simulink model "poco_ref_al_r307"  (Simulink 6.2)
settings: Solver=ode45  StartTime=0.0  StopTime=100000  RelTol=1e-3
libraries: xbsIndex_r3 x1012, xps_library x42, ddc_library x4, adcscope_lib x2, fft_library x2, pfb_library x2, delay_lib x1
(part 6 of 9)

== system poco_ref_al_r307/dir_x/bb ==
  a+bi : Inport  Port=1  LatchInput=off
  c+di : Inport  Port=2  LatchInput=off
  new_acc : Inport  Port=3  LatchInput=off
  Counter : xbsIndex_r3/Counter  cnt_type=Free Running  n_bits=11  bin_pt=0  arith_type=Unsigned  start_count=0  cnt_to=Inf  cnt_by_val=1  operation=Up  explicit_period=off  period=1  load_pin=off  rst=on  en=on  dbl_ovrd=off  show_param=off  use_rpm=on  gen_core=off
      settings: xl_area=[0, 0, 0, 0, 0, 0, 0]
  Delay3 : xbsIndex_r3/Delay  latency=5  reg_retiming=off  explicit_period=off  period=1  en=off  accept_only_valid=off  init_zero=on  dbl_ovrd=off  show_param=off
      settings: xl_area=[0, 0, 0, 0, 0, 0, 0]
  Reinterpret : xbsIndex_r3/Reinterpret  force_arith_type=on  arith_type=Unsigned  force_bin_pt=on  bin_pt=0  force_valid=on
  c_to_ri : Subsystem  mask(Complex to Real-Imag){n_bits=4, bin_pt=3}
      mask prompts: n_bits "Bit Width"; bin_pt "Binary Point"
      mask help: Outputs real and imaginary components of a complex input.
      mask init:
      | annotation=sprintf('%d_%d r/i',n_bits,bin_pt);
      | set_param(gcb,'AttributesFormatString',annotation);
      settings: AttributesFormatString=4_3 r/i
      mask Help:
      | <pre>
      | Description::
      | 
      | Outputs real and imaginary components of a complex input.
      | Useful for simplifying interconnects.
      | See also: Real-Imag to Complex (ri_to_c)
      | 
      | Mask Parameters::
      | 
      | Bit Width (n_bits): Specifies the width of the real/imaginary components.
      | Assumed equal for both components.
      | 
      | Binary Point (bin_pt): Specifies the binary point location in the real/imaginary components.
      | Assumed equal for both components.
      | </pre>
  c_to_ri1 : Subsystem  mask(Complex to Real-Imag){n_bits=4, bin_pt=3}
      mask prompts: n_bits "Bit Width"; bin_pt "Binary Point"
      mask help: Outputs real and imaginary components of a complex input.
      mask init:
      | annotation=sprintf('%d_%d r/i',n_bits,bin_pt);
      | set_param(gcb,'AttributesFormatString',annotation);
      settings: AttributesFormatString=4_3 r/i
      mask Help:
      | <pre>
      | Description::
      | 
      | Outputs real and imaginary components of a complex input.
      | Useful for simplifying interconnects.
      | See also: Real-Imag to Complex (ri_to_c)
      | 
      | Mask Parameters::
      | 
      | Bit Width (n_bits): Specifies the width of the real/imaginary components.
      | Assumed equal for both components.
      | 
      | Binary Point (bin_pt): Specifies the binary point location in the real/imaginary components.
      | Assumed equal for both components.
      | </pre>
  cmult_4bit_br* : Subsystem  mask(cmult_4bit_br*){mult_latency=3, add_latency=2}
      mask prompts: mult_latency "Mult Latency"; add_latency "Add Latency"
      mask help: Perform a conjugating complex multiplication (a+bi)(c-di)=(ac+bd)+(bc-ad)i. Implements the logic in Block RAM.
      mask Help: eval('xlWeb([getenv(''MLIB_ROOT''), ''\doc\html\sp_cmult_4bit_br_\sp_cmult_4bit_br_.html''])')
  real : xps_library/Shared BRAM  Tag=xps:bram  arith_type=Unsigned  addr_width=chan_bits+1  data_width=32  data_bin_pt=0  init_vals=0  sample_rate=1
  vacc_32bit : Subsystem  mask{n_chans=n_chans}
      mask prompts: n_chans "Number of channels"
      mask init:
      | chan_bits=ceil(log2(n_chans));
  wires:
  cmult_4bit_br*/1(real) -> vacc_32bit/1(din)
  new_acc/1 -> Delay3/1
  vacc_32bit/1(dout) -> Reinterpret/1
  c_to_ri/1(re) -> cmult_4bit_br*/1(a)
  c_to_ri/2(im) -> cmult_4bit_br*/2(b)
  c_to_ri1/1(re) -> cmult_4bit_br*/3(c)
  c_to_ri1/2(im) -> cmult_4bit_br*/4(d)
  a+bi/1 -> c_to_ri/1(c)
  c+di/1 -> c_to_ri1/1(c)
  Delay3/1 -> Counter/1, vacc_32bit/2(new_acc)
  vacc_32bit/2(valid) -> real/3, Counter/2
  Counter/1 -> real/1
  Reinterpret/1 -> real/2

== system poco_ref_al_r307/dir_x/bc ==
  a+bi : Inport  Port=1  LatchInput=off
  c+di : Inport  Port=2  LatchInput=off
  new_acc : Inport  Port=3  LatchInput=off
  Counter : xbsIndex_r3/Counter  cnt_type=Free Running  n_bits=11  bin_pt=0  arith_type=Unsigned  start_count=0  cnt_to=Inf  cnt_by_val=1  operation=Up  explicit_period=off  period=1  load_pin=off  rst=on  en=on  dbl_ovrd=off  show_param=off  use_rpm=on  gen_core=off
      settings: xl_area=[0, 0, 0, 0, 0, 0, 0]
  Delay3 : xbsIndex_r3/Delay  latency=5  reg_retiming=off  explicit_period=off  period=1  en=off  accept_only_valid=off  init_zero=on  dbl_ovrd=off  show_param=off
      settings: xl_area=[0, 0, 0, 0, 0, 0, 0]
  Reinterpret : xbsIndex_r3/Reinterpret  force_arith_type=on  arith_type=Unsigned  force_bin_pt=on  bin_pt=0  force_valid=on
  Reinterpret1 : xbsIndex_r3/Reinterpret  force_arith_type=on  arith_type=Unsigned  force_bin_pt=on  bin_pt=0  force_valid=on
  c_to_ri : Subsystem  mask(Complex to Real-Imag){n_bits=4, bin_pt=3}
      mask prompts: n_bits "Bit Width"; bin_pt "Binary Point"
      mask help: Outputs real and imaginary components of a complex input.
      mask init:
      | annotation=sprintf('%d_%d r/i',n_bits,bin_pt);
      | set_param(gcb,'AttributesFormatString',annotation);
      settings: AttributesFormatString=4_3 r/i
      mask Help:
      | <pre>
      | Description::
      | 
      | Outputs real and imaginary components of a complex input.
      | Useful for simplifying interconnects.
      | See also: Real-Imag to Complex (ri_to_c)
      | 
      | Mask Parameters::
      | 
      | Bit Width (n_bits): Specifies the width of the real/imaginary components.
      | Assumed equal for both components.
      | 
      | Binary Point (bin_pt): Specifies the binary point location in the real/imaginary components.
      | Assumed equal for both components.
      | </pre>
  c_to_ri1 : Subsystem  mask(Complex to Real-Imag){n_bits=4, bin_pt=3}
      mask prompts: n_bits "Bit Width"; bin_pt "Binary Point"
      mask help: Outputs real and imaginary components of a complex input.
      mask init:
      | annotation=sprintf('%d_%d r/i',n_bits,bin_pt);
      | set_param(gcb,'AttributesFormatString',annotation);
      settings: AttributesFormatString=4_3 r/i
      mask Help:
      | <pre>
      | Description::
      | 
      | Outputs real and imaginary components of a complex input.
      | Useful for simplifying interconnects.
      | See also: Real-Imag to Complex (ri_to_c)
      | 
      | Mask Parameters::
      | 
      | Bit Width (n_bits): Specifies the width of the real/imaginary components.
      | Assumed equal for both components.
      | 
      | Binary Point (bin_pt): Specifies the binary point location in the real/imaginary components.
      | Assumed equal for both components.
      | </pre>
  cmult_4bit_sl* : Subsystem  mask(cmult_4bit_sl*){mult_latency=3, add_latency=2}
      mask prompts: mult_latency "Mult Latency"; add_latency "Add Latency"
      mask help: Perform a conjugating complex multiplication (a+bi)(c-di)=(ac+bd)+(bc-ad)i. Implements the logic in Slices.
      mask Help: eval('xlWeb([getenv(''MLIB_ROOT''), ''\doc\html\sp_cmult_4bit_sl_\sp_cmult_4bit_sl_.html''])')
  imag : xps_library/Shared BRAM  Tag=xps:bram  arith_type=Unsigned  addr_width=chan_bits+1  data_width=32  data_bin_pt=0  init_vals=0  sample_rate=1
  real : xps_library/Shared BRAM  Tag=xps:bram  arith_type=Unsigned  addr_width=chan_bits+1  data_width=32  data_bin_pt=0  init_vals=0  sample_rate=1
  vacc_0 : Subsystem  mask{n_chans=n_chans}
      mask prompts: n_chans "Number of channels"
      mask init:
      | chan_bits=ceil(log2(n_chans));
  vacc_1 : Subsystem  mask{n_chans=n_chans}
      mask prompts: n_chans "Number of channels"
      mask init:
      | chan_bits=ceil(log2(n_chans));
  wires:
  Counter/1 -> real/1, imag/1
  vacc_1/1(dout) -> Reinterpret1/1
  Reinterpret1/1 -> imag/2
  vacc_1/2(valid) -> imag/3
  Reinterpret/1 -> real/2
  vacc_0/2(valid) -> real/3, Counter/2
  vacc_0/1(dout) -> Reinterpret/1
  new_acc/1 -> Delay3/1
  Delay3/1 -> Counter/1, vacc_0/2(new_acc), vacc_1/2(new_acc)
  c+di/1 -> c_to_ri1/1(c)
  a+bi/1 -> c_to_ri/1(c)
  c_to_ri1/2(im) -> cmult_4bit_sl*/4(d)
  c_to_ri1/1(re) -> cmult_4bit_sl*/3(c)
  c_to_ri/2(im) -> cmult_4bit_sl*/2(b)
  c_to_ri/1(re) -> cmult_4bit_sl*/1(a)
  cmult_4bit_sl*/2(imag) -> vacc_1/1(din)
  cmult_4bit_sl*/1(real) -> vacc_0/1(din)

== system poco_ref_al_r307/dir_x/bd ==
  a+bi : Inport  Port=1  LatchInput=off
  c+di : Inport  Port=2  LatchInput=off
  new_acc : Inport  Port=3  LatchInput=off
  Counter : xbsIndex_r3/Counter  cnt_type=Free Running  n_bits=11  bin_pt=0  arith_type=Unsigned  start_count=0  cnt_to=Inf  cnt_by_val=1  operation=Up  explicit_period=off  period=1  load_pin=off  rst=on  en=on  dbl_ovrd=off  show_param=off  use_rpm=on  gen_core=off
      settings: xl_area=[0, 0, 0, 0, 0, 0, 0]
  Delay3 : xbsIndex_r3/Delay  latency=5  reg_retiming=off  explicit_period=off  period=1  en=off  accept_only_valid=off  init_zero=on  dbl_ovrd=off  show_param=off
      settings: xl_area=[0, 0, 0, 0, 0, 0, 0]
  Reinterpret : xbsIndex_r3/Reinterpret  force_arith_type=on  arith_type=Unsigned  force_bin_pt=on  bin_pt=0  force_valid=on
  Reinterpret1 : xbsIndex_r3/Reinterpret  force_arith_type=on  arith_type=Unsigned  force_bin_pt=on  bin_pt=0  force_valid=on
  c_to_ri : Subsystem  mask(Complex to Real-Imag){n_bits=4, bin_pt=3}
      mask prompts: n_bits "Bit Width"; bin_pt "Binary Point"
      mask help: Outputs real and imaginary components of a complex input.
      mask init:
      | annotation=sprintf('%d_%d r/i',n_bits,bin_pt);
      | set_param(gcb,'AttributesFormatString',annotation);
      settings: AttributesFormatString=4_3 r/i
      mask Help:
      | <pre>
      | Description::
      | 
      | Outputs real and imaginary components of a complex input.
      | Useful for simplifying interconnects.
      | See also: Real-Imag to Complex (ri_to_c)
      | 
      | Mask Parameters::
      | 
      | Bit Width (n_bits): Specifies the width of the real/imaginary components.
      | Assumed equal for both components.
      | 
      | Binary Point (bin_pt): Specifies the binary point location in the real/imaginary components.
      | Assumed equal for both components.
      | </pre>
  c_to_ri1 : Subsystem  mask(Complex to Real-Imag){n_bits=4, bin_pt=3}
      mask prompts: n_bits "Bit Width"; bin_pt "Binary Point"
      mask help: Outputs real and imaginary components of a complex input.
      mask init:
      | annotation=sprintf('%d_%d r/i',n_bits,bin_pt);
      | set_param(gcb,'AttributesFormatString',annotation);
      settings: AttributesFormatString=4_3 r/i
      mask Help:
      | <pre>
      | Description::
      | 
      | Outputs real and imaginary components of a complex input.
      | Useful for simplifying interconnects.
      | See also: Real-Imag to Complex (ri_to_c)
      | 
      | Mask Parameters::
      | 
      | Bit Width (n_bits): Specifies the width of the real/imaginary components.
      | Assumed equal for both components.
      | 
      | Binary Point (bin_pt): Specifies the binary point location in the real/imaginary components.
      | Assumed equal for both components.
      | </pre>
  cmult_4bit_sl* : Subsystem  mask(cmult_4bit_sl*){mult_latency=3, add_latency=2}
      mask prompts: mult_latency "Mult Latency"; add_latency "Add Latency"
      mask help: Perform a conjugating complex multiplication (a+bi)(c-di)=(ac+bd)+(bc-ad)i. Implements the logic in Slices.
      mask Help: eval('xlWeb([getenv(''MLIB_ROOT''), ''\doc\html\sp_cmult_4bit_sl_\sp_cmult_4bit_sl_.html''])')
  imag : xps_library/Shared BRAM  Tag=xps:bram  arith_type=Unsigned  addr_width=chan_bits+1  data_width=32  data_bin_pt=0  init_vals=0  sample_rate=1
  real : xps_library/Shared BRAM  Tag=xps:bram  arith_type=Unsigned  addr_width=chan_bits+1  data_width=32  data_bin_pt=0  init_vals=0  sample_rate=1
  vacc_0 : Subsystem  mask{n_chans=n_chans}
      mask prompts: n_chans "Number of channels"
      mask init:
      | chan_bits=ceil(log2(n_chans));
  vacc_1 : Subsystem  mask{n_chans=n_chans}
      mask prompts: n_chans "Number of channels"
      mask init:
      | chan_bits=ceil(log2(n_chans));
  wires:
  cmult_4bit_sl*/1(real) -> vacc_0/1(din)
  cmult_4bit_sl*/2(imag) -> vacc_1/1(din)
  c_to_ri/1(re) -> cmult_4bit_sl*/1(a)
  c_to_ri/2(im) -> cmult_4bit_sl*/2(b)
  c_to_ri1/1(re) -> cmult_4bit_sl*/3(c)
  c_to_ri1/2(im) -> cmult_4bit_sl*/4(d)
  a+bi/1 -> c_to_ri/1(c)
  c+di/1 -> c_to_ri1/1(c)
  Delay3/1 -> Counter/1, vacc_0/2(new_acc), vacc_1/2(new_acc)
  new_acc/1 -> Delay3/1
  vacc_0/1(dout) -> Reinterpret/1
  vacc_0/2(valid) -> Counter/2, real/3
  Reinterpret/1 -> real/2
  vacc_1/2(valid) -> imag/3
  Reinterpret1/1 -> imag/2
  vacc_1/1(dout) -> Reinterpret1/1
  Counter/1 -> imag/1, real/1

== system poco_ref_al_r307/dir_x/cc ==
  a+bi : Inport  Port=1  LatchInput=off
  c+di : Inport  Port=2  LatchInput=off
  new_acc : Inport  Port=3  LatchInput=off
  Counter : xbsIndex_r3/Counter  cnt_type=Free Running  n_bits=11  bin_pt=0  arith_type=Unsigned  start_count=0  cnt_to=Inf  cnt_by_val=1  operation=Up  explicit_period=off  period=1  load_pin=off  rst=on  en=on  dbl_ovrd=off  show_param=off  use_rpm=on  gen_core=off
      settings: xl_area=[0, 0, 0, 0, 0, 0, 0]
  Delay3 : xbsIndex_r3/Delay  latency=5  reg_retiming=off  explicit_period=off  period=1  en=off  accept_only_valid=off  init_zero=on  dbl_ovrd=off  show_param=off
      settings: xl_area=[0, 0, 0, 0, 0, 0, 0]
  Reinterpret : xbsIndex_r3/Reinterpret  force_arith_type=on  arith_type=Unsigned  force_bin_pt=on  bin_pt=0  force_valid=on
  c_to_ri : Subsystem  mask(Complex to Real-Imag){n_bits=4, bin_pt=3}
      mask prompts: n_bits "Bit Width"; bin_pt "Binary Point"
      mask help: Outputs real and imaginary components of a complex input.
      mask init:
      | annotation=sprintf('%d_%d r/i',n_bits,bin_pt);
      | set_param(gcb,'AttributesFormatString',annotation);
      settings: AttributesFormatString=4_3 r/i
      mask Help:
      | <pre>
      | Description::
      | 
      | Outputs real and imaginary components of a complex input.
      | Useful for simplifying interconnects.
      | See also: Real-Imag to Complex (ri_to_c)
      | 
      | Mask Parameters::
      | 
      | Bit Width (n_bits): Specifies the width of the real/imaginary components.
      | Assumed equal for both components.
      | 
      | Binary Point (bin_pt): Specifies the binary point location in the real/imaginary components.
      | Assumed equal for both components.
      | </pre>
  c_to_ri1 : Subsystem  mask(Complex to Real-Imag){n_bits=4, bin_pt=3}
      mask prompts: n_bits "Bit Width"; bin_pt "Binary Point"
      mask help: Outputs real and imaginary components of a complex input.
      mask init:
      | annotation=sprintf('%d_%d r/i',n_bits,bin_pt);
      | set_param(gcb,'AttributesFormatString',annotation);
      settings: AttributesFormatString=4_3 r/i
      mask Help:
      | <pre>
      | Description::
      | 
      | Outputs real and imaginary components of a complex input.
      | Useful for simplifying interconnects.
      | See also: Real-Imag to Complex (ri_to_c)
      | 
      | Mask Parameters::
      | 
      | Bit Width (n_bits): Specifies the width of the real/imaginary components.
      | Assumed equal for both components.
      | 
      | Binary Point (bin_pt): Specifies the binary point location in the real/imaginary components.
      | Assumed equal for both components.
      | </pre>
  cmult_4bit_br* : Subsystem  mask(cmult_4bit_br*){mult_latency=3, add_latency=2}
      mask prompts: mult_latency "Mult Latency"; add_latency "Add Latency"
      mask help: Perform a conjugating complex multiplication (a+bi)(c-di)=(ac+bd)+(bc-ad)i. Implements the logic in Block RAM.
      mask Help: eval('xlWeb([getenv(''MLIB_ROOT''), ''\doc\html\sp_cmult_4bit_br_\sp_cmult_4bit_br_.html''])')
  real : xps_library/Shared BRAM  Tag=xps:bram  arith_type=Unsigned  addr_width=chan_bits+1  data_width=32  data_bin_pt=0  init_vals=0  sample_rate=1
  vacc_32bit : Subsystem  mask{n_chans=n_chans}
      mask prompts: n_chans "Number of channels"
      mask init:
      | chan_bits=ceil(log2(n_chans));
  wires:
  Reinterpret/1 -> real/2
  Counter/1 -> real/1
  vacc_32bit/2(valid) -> Counter/2, real/3
  Delay3/1 -> Counter/1, vacc_32bit/2(new_acc)
  c+di/1 -> c_to_ri1/1(c)
  a+bi/1 -> c_to_ri/1(c)
  c_to_ri1/2(im) -> cmult_4bit_br*/4(d)
  c_to_ri1/1(re) -> cmult_4bit_br*/3(c)
  c_to_ri/2(im) -> cmult_4bit_br*/2(b)
  c_to_ri/1(re) -> cmult_4bit_br*/1(a)
  vacc_32bit/1(dout) -> Reinterpret/1
  new_acc/1 -> Delay3/1
  cmult_4bit_br*/1(real) -> vacc_32bit/1(din)

== system poco_ref_al_r307/dir_x/cd ==
  a+bi : Inport  Port=1  LatchInput=off
  c+di : Inport  Port=2  LatchInput=off
  new_acc : Inport  Port=3  LatchInput=off
  Counter : xbsIndex_r3/Counter  cnt_type=Free Running  n_bits=11  bin_pt=0  arith_type=Unsigned  start_count=0  cnt_to=Inf  cnt_by_val=1  operation=Up  explicit_period=off  period=1  load_pin=off  rst=on  en=on  dbl_ovrd=off  show_param=off  use_rpm=on  gen_core=off
      settings: xl_area=[0, 0, 0, 0, 0, 0, 0]
  Delay3 : xbsIndex_r3/Delay  latency=5  reg_retiming=off  explicit_period=off  period=1  en=off  accept_only_valid=off  init_zero=on  dbl_ovrd=off  show_param=off
      settings: xl_area=[0, 0, 0, 0, 0, 0, 0]
  Reinterpret : xbsIndex_r3/Reinterpret  force_arith_type=on  arith_type=Unsigned  force_bin_pt=on  bin_pt=0  force_valid=on
  Reinterpret1 : xbsIndex_r3/Reinterpret  force_arith_type=on  arith_type=Unsigned  force_bin_pt=on  bin_pt=0  force_valid=on
  c_to_ri : Subsystem  mask(Complex to Real-Imag){n_bits=4, bin_pt=3}
      mask prompts: n_bits "Bit Width"; bin_pt "Binary Point"
      mask help: Outputs real and imaginary components of a complex input.
      mask init:
      | annotation=sprintf('%d_%d r/i',n_bits,bin_pt);
      | set_param(gcb,'AttributesFormatString',annotation);
      settings: AttributesFormatString=4_3 r/i
      mask Help:
      | <pre>
      | Description::
      | 
      | Outputs real and imaginary components of a complex input.
      | Useful for simplifying interconnects.
      | See also: Real-Imag to Complex (ri_to_c)
      | 
      | Mask Parameters::
      | 
      | Bit Width (n_bits): Specifies the width of the real/imaginary components.
      | Assumed equal for both components.
      | 
      | Binary Point (bin_pt): Specifies the binary point location in the real/imaginary components.
      | Assumed equal for both components.
      | </pre>
  c_to_ri1 : Subsystem  mask(Complex to Real-Imag){n_bits=4, bin_pt=3}
      mask prompts: n_bits "Bit Width"; bin_pt "Binary Point"
      mask help: Outputs real and imaginary components of a complex input.
      mask init:
      | annotation=sprintf('%d_%d r/i',n_bits,bin_pt);
      | set_param(gcb,'AttributesFormatString',annotation);
      settings: AttributesFormatString=4_3 r/i
      mask Help:
      | <pre>
      | Description::
      | 
      | Outputs real and imaginary components of a complex input.
      | Useful for simplifying interconnects.
      | See also: Real-Imag to Complex (ri_to_c)
      | 
      | Mask Parameters::
      | 
      | Bit Width (n_bits): Specifies the width of the real/imaginary components.
      | Assumed equal for both components.
      | 
      | Binary Point (bin_pt): Specifies the binary point location in the real/imaginary components.
      | Assumed equal for both components.
      | </pre>
  cmult_4bit_sl* : Subsystem  mask(cmult_4bit_sl*){mult_latency=3, add_latency=2}
      mask prompts: mult_latency "Mult Latency"; add_latency "Add Latency"
      mask help: Perform a conjugating complex multiplication (a+bi)(c-di)=(ac+bd)+(bc-ad)i. Implements the logic in Slices.
      mask Help: eval('xlWeb([getenv(''MLIB_ROOT''), ''\doc\html\sp_cmult_4bit_sl_\sp_cmult_4bit_sl_.html''])')
  imag : xps_library/Shared BRAM  Tag=xps:bram  arith_type=Unsigned  addr_width=chan_bits+1  data_width=32  data_bin_pt=0  init_vals=0  sample_rate=1
  real : xps_library/Shared BRAM  Tag=xps:bram  arith_type=Unsigned  addr_width=chan_bits+1  data_width=32  data_bin_pt=0  init_vals=0  sample_rate=1
  vacc_0 : Subsystem  mask{n_chans=n_chans}
      mask prompts: n_chans "Number of channels"
      mask init:
      | chan_bits=ceil(log2(n_chans));
  vacc_1 : Subsystem  mask{n_chans=n_chans}
      mask prompts: n_chans "Number of channels"
      mask init:
      | chan_bits=ceil(log2(n_chans));
  wires:
  Counter/1 -> real/1, imag/1
  vacc_1/1(dout) -> Reinterpret1/1
  Reinterpret1/1 -> imag/2
  vacc_1/2(valid) -> imag/3
  Reinterpret/1 -> real/2
  vacc_0/2(valid) -> real/3, Counter/2
  vacc_0/1(dout) -> Reinterpret/1
  new_acc/1 -> Delay3/1
  Delay3/1 -> Counter/1, vacc_0/2(new_acc), vacc_1/2(new_acc)
  c+di/1 -> c_to_ri1/1(c)
  a+bi/1 -> c_to_ri/1(c)
  c_to_ri1/2(im) -> cmult_4bit_sl*/4(d)
  c_to_ri1/1(re) -> cmult_4bit_sl*/3(c)
  c_to_ri/2(im) -> cmult_4bit_sl*/2(b)
  c_to_ri/1(re) -> cmult_4bit_sl*/1(a)
  cmult_4bit_sl*/2(imag) -> vacc_1/1(din)
  cmult_4bit_sl*/1(real) -> vacc_0/1(din)

== system poco_ref_al_r307/dir_x/dd ==
  a+bi : Inport  Port=1  LatchInput=off
  c+di : Inport  Port=2  LatchInput=off
  new_acc : Inport  Port=3  LatchInput=off
  Counter : xbsIndex_r3/Counter  cnt_type=Free Running  n_bits=11  bin_pt=0  arith_type=Unsigned  start_count=0  cnt_to=Inf  cnt_by_val=1  operation=Up  explicit_period=off  period=1  load_pin=off  rst=on  en=on  dbl_ovrd=off  show_param=off  use_rpm=on  gen_core=off
      settings: xl_area=[0, 0, 0, 0, 0, 0, 0]
  Delay3 : xbsIndex_r3/Delay  latency=5  reg_retiming=off  explicit_period=off  period=1  en=off  accept_only_valid=off  init_zero=on  dbl_ovrd=off  show_param=off
      settings: xl_area=[0, 0, 0, 0, 0, 0, 0]
  Reinterpret : xbsIndex_r3/Reinterpret  force_arith_type=on  arith_type=Unsigned  force_bin_pt=on  bin_pt=0  force_valid=on
  c_to_ri : Subsystem  mask(Complex to Real-Imag){n_bits=4, bin_pt=3}
      mask prompts: n_bits "Bit Width"; bin_pt "Binary Point"
      mask help: Outputs real and imaginary components of a complex input.
      mask init:
      | annotation=sprintf('%d_%d r/i',n_bits,bin_pt);
      | set_param(gcb,'AttributesFormatString',annotation);
      settings: AttributesFormatString=4_3 r/i
      mask Help:
      | <pre>
      | Description::
      | 
      | Outputs real and imaginary components of a complex input.
      | Useful for simplifying interconnects.
      | See also: Real-Imag to Complex (ri_to_c)
      | 
      | Mask Parameters::
      | 
      | Bit Width (n_bits): Specifies the width of the real/imaginary components.
      | Assumed equal for both components.
      | 
      | Binary Point (bin_pt): Specifies the binary point location in the real/imaginary components.
      | Assumed equal for both components.
      | </pre>
  c_to_ri1 : Subsystem  mask(Complex to Real-Imag){n_bits=4, bin_pt=3}
      mask prompts: n_bits "Bit Width"; bin_pt "Binary Point"
      mask help: Outputs real and imaginary components of a complex input.
      mask init:
      | annotation=sprintf('%d_%d r/i',n_bits,bin_pt);
      | set_param(gcb,'AttributesFormatString',annotation);
      settings: AttributesFormatString=4_3 r/i
      mask Help:
      | <pre>
      | Description::
      | 
      | Outputs real and imaginary components of a complex input.
      | Useful for simplifying interconnects.
      | See also: Real-Imag to Complex (ri_to_c)
      | 
      | Mask Parameters::
      | 
      | Bit Width (n_bits): Specifies the width of the real/imaginary components.
      | Assumed equal for both components.
      | 
      | Binary Point (bin_pt): Specifies the binary point location in the real/imaginary components.
      | Assumed equal for both components.
      | </pre>
  cmult_4bit_br* : Subsystem  mask(cmult_4bit_br*){mult_latency=3, add_latency=2}
      mask prompts: mult_latency "Mult Latency"; add_latency "Add Latency"
      mask help: Perform a conjugating complex multiplication (a+bi)(c-di)=(ac+bd)+(bc-ad)i. Implements the logic in Block RAM.
      mask Help: eval('xlWeb([getenv(''MLIB_ROOT''), ''\doc\html\sp_cmult_4bit_br_\sp_cmult_4bit_br_.html''])')
  real : xps_library/Shared BRAM  Tag=xps:bram  arith_type=Unsigned  addr_width=chan_bits+1  data_width=32  data_bin_pt=0  init_vals=0  sample_rate=1
  vacc_32bit : Subsystem  mask{n_chans=n_chans}
      mask prompts: n_chans "Number of channels"
      mask init:
      | chan_bits=ceil(log2(n_chans));
  wires:
  cmult_4bit_br*/1(real) -> vacc_32bit/1(din)
  new_acc/1 -> Delay3/1
  vacc_32bit/1(dout) -> Reinterpret/1
  c_to_ri/1(re) -> cmult_4bit_br*/1(a)
  c_to_ri/2(im) -> cmult_4bit_br*/2(b)
  c_to_ri1/1(re) -> cmult_4bit_br*/3(c)
  c_to_ri1/2(im) -> cmult_4bit_br*/4(d)
  a+bi/1 -> c_to_ri/1(c)
  c+di/1 -> c_to_ri1/1(c)
  Delay3/1 -> Counter/1, vacc_32bit/2(new_acc)
  vacc_32bit/2(valid) -> real/3, Counter/2
  Counter/1 -> real/1
  Reinterpret/1 -> real/2

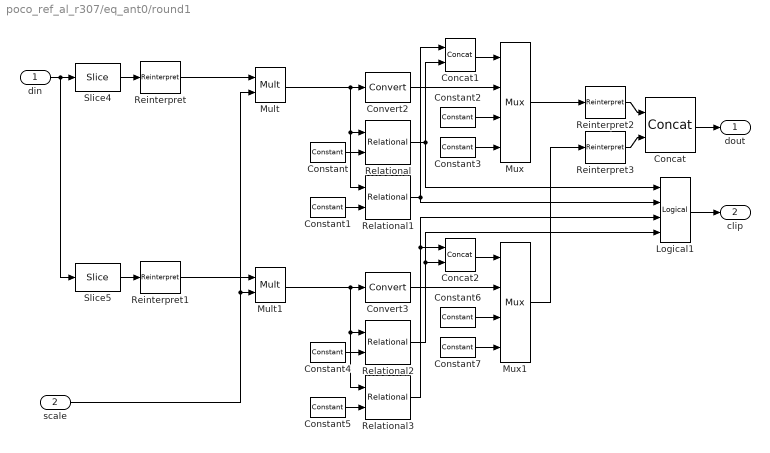
== system poco_ref_al_r307/eq_ant0/round1 ==
  din : Inport  Port=1  LatchInput=off
  scale : Inport  Port=2  LatchInput=off
  Concat : xbsIndex_r3/Concat  num_inputs=2  explicit_period=off  period=1  dbl_ovrd=off
  Concat1 : xbsIndex_r3/Concat  num_inputs=2  explicit_period=off  period=1  dbl_ovrd=off
  Concat2 : xbsIndex_r3/Concat  num_inputs=2  explicit_period=off  period=1  dbl_ovrd=off
  Constant : xbsIndex_r3/Constant  const=7/8  equ=P=C  arith_type="Signed  (2's comp)"  n_bits=27  bin_pt=18  opselect=C  inp2=PCIN>>17  opr=+  inp1=P  carry=CIN  iostate=0  explicit_period=on  period=1  dbl_ovrd=off
  Constant1 : xbsIndex_r3/Constant  const=-7/8  equ=P=C  arith_type="Signed  (2's comp)"  n_bits=27  bin_pt=18  opselect=C  inp2=PCIN>>17  opr=+  inp1=P  carry=CIN  iostate=0  explicit_period=on  period=1  dbl_ovrd=off
  Constant2 : xbsIndex_r3/Constant  const=7/8  equ=P=C  arith_type="Signed  (2's comp)"  n_bits=4  bin_pt=3  opselect=C  inp2=PCIN>>17  opr=+  inp1=P  carry=CIN  iostate=0  explicit_period=on  period=1  dbl_ovrd=off
  Constant3 : xbsIndex_r3/Constant  const=-7/8  equ=P=C  arith_type="Signed  (2's comp)"  n_bits=4  bin_pt=3  opselect=C  inp2=PCIN>>17  opr=+  inp1=P  carry=CIN  iostate=0  explicit_period=on  period=1  dbl_ovrd=off
  Constant4 : xbsIndex_r3/Constant  const=7/8  equ=P=C  arith_type="Signed  (2's comp)"  n_bits=27  bin_pt=18  opselect=C  inp2=PCIN>>17  opr=+  inp1=P  carry=CIN  iostate=0  explicit_period=on  period=1  dbl_ovrd=off
  Constant5 : xbsIndex_r3/Constant  const=-7/8  equ=P=C  arith_type="Signed  (2's comp)"  n_bits=27  bin_pt=18  opselect=C  inp2=PCIN>>17  opr=+  inp1=P  carry=CIN  iostate=0  explicit_period=on  period=1  dbl_ovrd=off
  Constant6 : xbsIndex_r3/Constant  const=7/8  equ=P=C  arith_type="Signed  (2's comp)"  n_bits=4  bin_pt=3  opselect=C  inp2=PCIN>>17  opr=+  inp1=P  carry=CIN  iostate=0  explicit_period=on  period=1  dbl_ovrd=off
  Constant7 : xbsIndex_r3/Constant  const=-7/8  equ=P=C  arith_type="Signed  (2's comp)"  n_bits=4  bin_pt=3  opselect=C  inp2=PCIN>>17  opr=+  inp1=P  carry=CIN  iostate=0  explicit_period=on  period=1  dbl_ovrd=off
  Convert2 : xbsIndex_r3/Convert  arith_type="Signed  (2's comp)"  n_bits=4  bin_pt=3  quantization="Round  (unbiased: Even Values)"  overflow=Wrap  latency=2  explicit_period=off  period=1  dbl_ovrd=off  show_param=off  inserted_by_tool=off  pipeline=off
      settings: xl_area=[0, 0, 0, 0, 0, 0, 0]
  Convert3 : xbsIndex_r3/Convert  arith_type="Signed  (2's comp)"  n_bits=4  bin_pt=3  quantization="Round  (unbiased: Even Values)"  overflow=Wrap  latency=2  explicit_period=off  period=1  dbl_ovrd=off  show_param=off  inserted_by_tool=off  pipeline=off
      settings: xl_area=[0, 0, 0, 0, 0, 0, 0]
  Logical1 : xbsIndex_r3/Logical  logical_function=OR  inputs=4  precision=Full  arith_type=Unsigned  n_bits=8  bin_pt=2  align_bp=on  latency=2  explicit_period=off  period=1  en=off  dbl_ovrd=off  show_param=off
      settings: xl_area=[0, 0, 0, 0, 0, 0, 0]
  Mult : xbsIndex_r3/Mult  precision=Full  arith_type="Signed  (2's comp)"  n_bits=8  bin_pt=2  quantization=Truncate  overflow=Wrap  latency=2  explicit_period=off  period=1  en=off  dbl_ovrd=off  show_param=on  mult_type=Parallel  oversample=2  use_embedded=on  pipeline=on  use_rpm=on  placement_style=Rectangular Shape  gen_core=off
      settings: xl_area=[0, 0, 0, 0, 0, 0, 0]
  Mult1 : xbsIndex_r3/Mult  precision=Full  arith_type="Signed  (2's comp)"  n_bits=8  bin_pt=2  quantization=Truncate  overflow=Wrap  latency=2  explicit_period=off  period=1  en=off  dbl_ovrd=off  show_param=on  mult_type=Parallel  oversample=2  use_embedded=on  pipeline=on  use_rpm=on  placement_style=Rectangular Shape  gen_core=off
      settings: xl_area=[0, 0, 0, 0, 0, 0, 0]
  Mux : xbsIndex_r3/Mux  inputs=3  precision=Full  arith_type="Signed  (2's comp)"  n_bits=8  bin_pt=2  quantization=Truncate  overflow=Wrap  latency=0  explicit_period=off  period=1  en=off  dbl_ovrd=off  show_param=off  mux_type=off  use_rpm=off  gen_core=off
      settings: xl_area=[0, 0, 0, 0, 0, 0, 0]
  Mux1 : xbsIndex_r3/Mux  inputs=3  precision=Full  arith_type="Signed  (2's comp)"  n_bits=8  bin_pt=2  quantization=Truncate  overflow=Wrap  latency=0  explicit_period=off  period=1  en=off  dbl_ovrd=off  show_param=off  mux_type=off  use_rpm=off  gen_core=off
      settings: xl_area=[0, 0, 0, 0, 0, 0, 0]
  Reinterpret : xbsIndex_r3/Reinterpret  force_arith_type=on  arith_type="Signed  (2's comp)"  force_bin_pt=on  bin_pt=17  force_valid=on
  Reinterpret1 : xbsIndex_r3/Reinterpret  force_arith_type=on  arith_type="Signed  (2's comp)"  force_bin_pt=on  bin_pt=17  force_valid=on
  Reinterpret2 : xbsIndex_r3/Reinterpret  force_arith_type=on  arith_type=Unsigned  force_bin_pt=on  bin_pt=0  force_valid=on
  Reinterpret3 : xbsIndex_r3/Reinterpret  force_arith_type=on  arith_type=Unsigned  force_bin_pt=on  bin_pt=0  force_valid=on
  Relational : xbsIndex_r3/Relational  mode=a>b  latency=2  explicit_period=off  period=1  en=off  dbl_ovrd=off  show_param=off
      settings: xl_area=[0, 0, 0, 0, 0, 0, 0]
  Relational1 : xbsIndex_r3/Relational  mode=a<b  latency=2  explicit_period=off  period=1  en=off  dbl_ovrd=off  show_param=off
      settings: xl_area=[0, 0, 0, 0, 0, 0, 0]
  Relational2 : xbsIndex_r3/Relational  mode=a>b  latency=2  explicit_period=off  period=1  en=off  dbl_ovrd=off  show_param=off
      settings: xl_area=[0, 0, 0, 0, 0, 0, 0]
  Relational3 : xbsIndex_r3/Relational  mode=a<b  latency=2  explicit_period=off  period=1  en=off  dbl_ovrd=off  show_param=off
      settings: xl_area=[0, 0, 0, 0, 0, 0, 0]
  Slice4 : xbsIndex_r3/Slice  mode=Upper Bit Location + Width  nbits=18  bit1=0  base1=MSB of Input  bit0=0  base0=LSB of Input  boolean_output=off  explicit_period=off  period=1  dbl_ovrd=off
  Slice5 : xbsIndex_r3/Slice  mode=Lower Bit Location + Width  nbits=18  bit1=0  base1=MSB of Input  bit0=0  base0=LSB of Input  boolean_output=off  explicit_period=off  period=1  dbl_ovrd=off
  dout : Outport
  clip : Outport  Port=2
  wires:
  Slice4/1 -> Reinterpret/1
  Reinterpret2/1 -> Concat/1
  Slice5/1 -> Reinterpret1/1
  Reinterpret3/1 -> Concat/2
  din/1 -> Slice4/1, Slice5/1
  Concat/1 -> dout/1
  Reinterpret1/1 -> Mult1/1
  Reinterpret/1 -> Mult/1
  scale/1 -> Mult1/2, Mult/2
  Convert2/1 -> Mux/2
  Concat1/1 -> Mux/1
  Constant/1 -> Relational/2
  Constant1/1 -> Relational1/2
  Constant2/1 -> Mux/3
  Constant3/1 -> Mux/4
  Relational/1 -> Concat1/2, Logical1/1
  Relational1/1 -> Concat1/1, Logical1/2
  Convert3/1 -> Mux1/2
  Concat2/1 -> Mux1/1
  Constant4/1 -> Relational2/2
  Constant5/1 -> Relational3/2
  Constant6/1 -> Mux1/3
  Constant7/1 -> Mux1/4
  Relational2/1 -> Concat2/2, Logical1/4
  Relational3/1 -> Concat2/1, Logical1/3
  Mux/1 -> Reinterpret2/1
  Mux1/1 -> Reinterpret3/1
  Mult1/1 -> Convert3/1, Relational2/1, Relational3/1
  Mult/1 -> Convert2/1, Relational/1, Relational1/1
  Logical1/1 -> clip/1

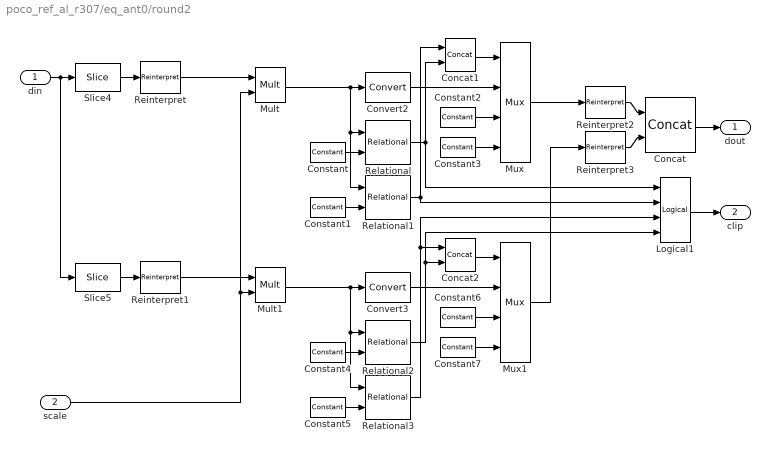
== system poco_ref_al_r307/eq_ant0/round2 ==
  din : Inport  Port=1  LatchInput=off
  scale : Inport  Port=2  LatchInput=off
  Concat : xbsIndex_r3/Concat  num_inputs=2  explicit_period=off  period=1  dbl_ovrd=off
  Concat1 : xbsIndex_r3/Concat  num_inputs=2  explicit_period=off  period=1  dbl_ovrd=off
  Concat2 : xbsIndex_r3/Concat  num_inputs=2  explicit_period=off  period=1  dbl_ovrd=off
  Constant : xbsIndex_r3/Constant  const=7/8  equ=P=C  arith_type="Signed  (2's comp)"  n_bits=27  bin_pt=18  opselect=C  inp2=PCIN>>17  opr=+  inp1=P  carry=CIN  iostate=0  explicit_period=on  period=1  dbl_ovrd=off
  Constant1 : xbsIndex_r3/Constant  const=-7/8  equ=P=C  arith_type="Signed  (2's comp)"  n_bits=27  bin_pt=18  opselect=C  inp2=PCIN>>17  opr=+  inp1=P  carry=CIN  iostate=0  explicit_period=on  period=1  dbl_ovrd=off
  Constant2 : xbsIndex_r3/Constant  const=7/8  equ=P=C  arith_type="Signed  (2's comp)"  n_bits=4  bin_pt=3  opselect=C  inp2=PCIN>>17  opr=+  inp1=P  carry=CIN  iostate=0  explicit_period=on  period=1  dbl_ovrd=off
  Constant3 : xbsIndex_r3/Constant  const=-7/8  equ=P=C  arith_type="Signed  (2's comp)"  n_bits=4  bin_pt=3  opselect=C  inp2=PCIN>>17  opr=+  inp1=P  carry=CIN  iostate=0  explicit_period=on  period=1  dbl_ovrd=off
  Constant4 : xbsIndex_r3/Constant  const=7/8  equ=P=C  arith_type="Signed  (2's comp)"  n_bits=27  bin_pt=18  opselect=C  inp2=PCIN>>17  opr=+  inp1=P  carry=CIN  iostate=0  explicit_period=on  period=1  dbl_ovrd=off
  Constant5 : xbsIndex_r3/Constant  const=-7/8  equ=P=C  arith_type="Signed  (2's comp)"  n_bits=27  bin_pt=18  opselect=C  inp2=PCIN>>17  opr=+  inp1=P  carry=CIN  iostate=0  explicit_period=on  period=1  dbl_ovrd=off
  Constant6 : xbsIndex_r3/Constant  const=7/8  equ=P=C  arith_type="Signed  (2's comp)"  n_bits=4  bin_pt=3  opselect=C  inp2=PCIN>>17  opr=+  inp1=P  carry=CIN  iostate=0  explicit_period=on  period=1  dbl_ovrd=off
  Constant7 : xbsIndex_r3/Constant  const=-7/8  equ=P=C  arith_type="Signed  (2's comp)"  n_bits=4  bin_pt=3  opselect=C  inp2=PCIN>>17  opr=+  inp1=P  carry=CIN  iostate=0  explicit_period=on  period=1  dbl_ovrd=off
  Convert2 : xbsIndex_r3/Convert  arith_type="Signed  (2's comp)"  n_bits=4  bin_pt=3  quantization="Round  (unbiased: Even Values)"  overflow=Wrap  latency=2  explicit_period=off  period=1  dbl_ovrd=off  show_param=off  inserted_by_tool=off  pipeline=off
      settings: xl_area=[0, 0, 0, 0, 0, 0, 0]
  Convert3 : xbsIndex_r3/Convert  arith_type="Signed  (2's comp)"  n_bits=4  bin_pt=3  quantization="Round  (unbiased: Even Values)"  overflow=Wrap  latency=2  explicit_period=off  period=1  dbl_ovrd=off  show_param=off  inserted_by_tool=off  pipeline=off
      settings: xl_area=[0, 0, 0, 0, 0, 0, 0]
  Logical1 : xbsIndex_r3/Logical  logical_function=OR  inputs=4  precision=Full  arith_type=Unsigned  n_bits=8  bin_pt=2  align_bp=on  latency=2  explicit_period=off  period=1  en=off  dbl_ovrd=off  show_param=off
      settings: xl_area=[0, 0, 0, 0, 0, 0, 0]
  Mult : xbsIndex_r3/Mult  precision=Full  arith_type="Signed  (2's comp)"  n_bits=8  bin_pt=2  quantization=Truncate  overflow=Wrap  latency=2  explicit_period=off  period=1  en=off  dbl_ovrd=off  show_param=on  mult_type=Parallel  oversample=2  use_embedded=on  pipeline=on  use_rpm=on  placement_style=Rectangular Shape  gen_core=off
      settings: xl_area=[0, 0, 0, 0, 0, 0, 0]
  Mult1 : xbsIndex_r3/Mult  precision=Full  arith_type="Signed  (2's comp)"  n_bits=8  bin_pt=2  quantization=Truncate  overflow=Wrap  latency=2  explicit_period=off  period=1  en=off  dbl_ovrd=off  show_param=on  mult_type=Parallel  oversample=2  use_embedded=on  pipeline=on  use_rpm=on  placement_style=Rectangular Shape  gen_core=off
      settings: xl_area=[0, 0, 0, 0, 0, 0, 0]
  Mux : xbsIndex_r3/Mux  inputs=3  precision=Full  arith_type="Signed  (2's comp)"  n_bits=8  bin_pt=2  quantization=Truncate  overflow=Wrap  latency=0  explicit_period=off  period=1  en=off  dbl_ovrd=off  show_param=off  mux_type=off  use_rpm=off  gen_core=off
      settings: xl_area=[0, 0, 0, 0, 0, 0, 0]
  Mux1 : xbsIndex_r3/Mux  inputs=3  precision=Full  arith_type="Signed  (2's comp)"  n_bits=8  bin_pt=2  quantization=Truncate  overflow=Wrap  latency=0  explicit_period=off  period=1  en=off  dbl_ovrd=off  show_param=off  mux_type=off  use_rpm=off  gen_core=off
      settings: xl_area=[0, 0, 0, 0, 0, 0, 0]
  Reinterpret : xbsIndex_r3/Reinterpret  force_arith_type=on  arith_type="Signed  (2's comp)"  force_bin_pt=on  bin_pt=17  force_valid=on
  Reinterpret1 : xbsIndex_r3/Reinterpret  force_arith_type=on  arith_type="Signed  (2's comp)"  force_bin_pt=on  bin_pt=17  force_valid=on
  Reinterpret2 : xbsIndex_r3/Reinterpret  force_arith_type=on  arith_type=Unsigned  force_bin_pt=on  bin_pt=0  force_valid=on
  Reinterpret3 : xbsIndex_r3/Reinterpret  force_arith_type=on  arith_type=Unsigned  force_bin_pt=on  bin_pt=0  force_valid=on
  Relational : xbsIndex_r3/Relational  mode=a>b  latency=2  explicit_period=off  period=1  en=off  dbl_ovrd=off  show_param=off
      settings: xl_area=[0, 0, 0, 0, 0, 0, 0]
  Relational1 : xbsIndex_r3/Relational  mode=a<b  latency=2  explicit_period=off  period=1  en=off  dbl_ovrd=off  show_param=off
      settings: xl_area=[0, 0, 0, 0, 0, 0, 0]
  Relational2 : xbsIndex_r3/Relational  mode=a>b  latency=2  explicit_period=off  period=1  en=off  dbl_ovrd=off  show_param=off
      settings: xl_area=[0, 0, 0, 0, 0, 0, 0]
  Relational3 : xbsIndex_r3/Relational  mode=a<b  latency=2  explicit_period=off  period=1  en=off  dbl_ovrd=off  show_param=off
      settings: xl_area=[0, 0, 0, 0, 0, 0, 0]
  Slice4 : xbsIndex_r3/Slice  mode=Upper Bit Location + Width  nbits=18  bit1=0  base1=MSB of Input  bit0=0  base0=LSB of Input  boolean_output=off  explicit_period=off  period=1  dbl_ovrd=off
  Slice5 : xbsIndex_r3/Slice  mode=Lower Bit Location + Width  nbits=18  bit1=0  base1=MSB of Input  bit0=0  base0=LSB of Input  boolean_output=off  explicit_period=off  period=1  dbl_ovrd=off
  dout : Outport
  clip : Outport  Port=2
  wires:
  Slice4/1 -> Reinterpret/1
  Reinterpret2/1 -> Concat/1
  Slice5/1 -> Reinterpret1/1
  Reinterpret3/1 -> Concat/2
  din/1 -> Slice4/1, Slice5/1
  Concat/1 -> dout/1
  Reinterpret1/1 -> Mult1/1
  Reinterpret/1 -> Mult/1
  scale/1 -> Mult1/2, Mult/2
  Convert2/1 -> Mux/2
  Concat1/1 -> Mux/1
  Constant/1 -> Relational/2
  Constant1/1 -> Relational1/2
  Constant2/1 -> Mux/3
  Constant3/1 -> Mux/4
  Relational/1 -> Concat1/2, Logical1/1
  Relational1/1 -> Concat1/1, Logical1/2
  Convert3/1 -> Mux1/2
  Concat2/1 -> Mux1/1
  Constant4/1 -> Relational2/2
  Constant5/1 -> Relational3/2
  Constant6/1 -> Mux1/3
  Constant7/1 -> Mux1/4
  Relational2/1 -> Concat2/2, Logical1/4
  Relational3/1 -> Concat2/1, Logical1/3
  Mux/1 -> Reinterpret2/1
  Mux1/1 -> Reinterpret3/1
  Mult1/1 -> Convert3/1, Relational2/1, Relational3/1
  Mult/1 -> Convert2/1, Relational/1, Relational1/1
  Logical1/1 -> clip/1

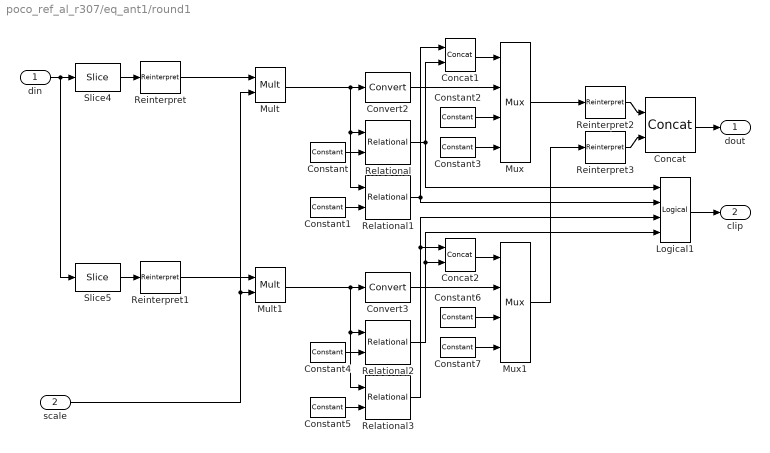
== system poco_ref_al_r307/eq_ant1/round1 ==
  din : Inport  Port=1  LatchInput=off
  scale : Inport  Port=2  LatchInput=off
  Concat : xbsIndex_r3/Concat  num_inputs=2  explicit_period=off  period=1  dbl_ovrd=off
  Concat1 : xbsIndex_r3/Concat  num_inputs=2  explicit_period=off  period=1  dbl_ovrd=off
  Concat2 : xbsIndex_r3/Concat  num_inputs=2  explicit_period=off  period=1  dbl_ovrd=off
  Constant : xbsIndex_r3/Constant  const=7/8  equ=P=C  arith_type="Signed  (2's comp)"  n_bits=27  bin_pt=18  opselect=C  inp2=PCIN>>17  opr=+  inp1=P  carry=CIN  iostate=0  explicit_period=on  period=1  dbl_ovrd=off
  Constant1 : xbsIndex_r3/Constant  const=-7/8  equ=P=C  arith_type="Signed  (2's comp)"  n_bits=27  bin_pt=18  opselect=C  inp2=PCIN>>17  opr=+  inp1=P  carry=CIN  iostate=0  explicit_period=on  period=1  dbl_ovrd=off
  Constant2 : xbsIndex_r3/Constant  const=7/8  equ=P=C  arith_type="Signed  (2's comp)"  n_bits=4  bin_pt=3  opselect=C  inp2=PCIN>>17  opr=+  inp1=P  carry=CIN  iostate=0  explicit_period=on  period=1  dbl_ovrd=off
  Constant3 : xbsIndex_r3/Constant  const=-7/8  equ=P=C  arith_type="Signed  (2's comp)"  n_bits=4  bin_pt=3  opselect=C  inp2=PCIN>>17  opr=+  inp1=P  carry=CIN  iostate=0  explicit_period=on  period=1  dbl_ovrd=off
  Constant4 : xbsIndex_r3/Constant  const=7/8  equ=P=C  arith_type="Signed  (2's comp)"  n_bits=27  bin_pt=18  opselect=C  inp2=PCIN>>17  opr=+  inp1=P  carry=CIN  iostate=0  explicit_period=on  period=1  dbl_ovrd=off
  Constant5 : xbsIndex_r3/Constant  const=-7/8  equ=P=C  arith_type="Signed  (2's comp)"  n_bits=27  bin_pt=18  opselect=C  inp2=PCIN>>17  opr=+  inp1=P  carry=CIN  iostate=0  explicit_period=on  period=1  dbl_ovrd=off
  Constant6 : xbsIndex_r3/Constant  const=7/8  equ=P=C  arith_type="Signed  (2's comp)"  n_bits=4  bin_pt=3  opselect=C  inp2=PCIN>>17  opr=+  inp1=P  carry=CIN  iostate=0  explicit_period=on  period=1  dbl_ovrd=off
  Constant7 : xbsIndex_r3/Constant  const=-7/8  equ=P=C  arith_type="Signed  (2's comp)"  n_bits=4  bin_pt=3  opselect=C  inp2=PCIN>>17  opr=+  inp1=P  carry=CIN  iostate=0  explicit_period=on  period=1  dbl_ovrd=off
  Convert2 : xbsIndex_r3/Convert  arith_type="Signed  (2's comp)"  n_bits=4  bin_pt=3  quantization="Round  (unbiased: Even Values)"  overflow=Wrap  latency=2  explicit_period=off  period=1  dbl_ovrd=off  show_param=off  inserted_by_tool=off  pipeline=off
      settings: xl_area=[0, 0, 0, 0, 0, 0, 0]
  Convert3 : xbsIndex_r3/Convert  arith_type="Signed  (2's comp)"  n_bits=4  bin_pt=3  quantization="Round  (unbiased: Even Values)"  overflow=Wrap  latency=2  explicit_period=off  period=1  dbl_ovrd=off  show_param=off  inserted_by_tool=off  pipeline=off
      settings: xl_area=[0, 0, 0, 0, 0, 0, 0]
  Logical1 : xbsIndex_r3/Logical  logical_function=OR  inputs=4  precision=Full  arith_type=Unsigned  n_bits=8  bin_pt=2  align_bp=on  latency=2  explicit_period=off  period=1  en=off  dbl_ovrd=off  show_param=off
      settings: xl_area=[0, 0, 0, 0, 0, 0, 0]
  Mult : xbsIndex_r3/Mult  precision=Full  arith_type="Signed  (2's comp)"  n_bits=8  bin_pt=2  quantization=Truncate  overflow=Wrap  latency=2  explicit_period=off  period=1  en=off  dbl_ovrd=off  show_param=on  mult_type=Parallel  oversample=2  use_embedded=on  pipeline=on  use_rpm=on  placement_style=Rectangular Shape  gen_core=off
      settings: xl_area=[0, 0, 0, 0, 0, 0, 0]
  Mult1 : xbsIndex_r3/Mult  precision=Full  arith_type="Signed  (2's comp)"  n_bits=8  bin_pt=2  quantization=Truncate  overflow=Wrap  latency=2  explicit_period=off  period=1  en=off  dbl_ovrd=off  show_param=on  mult_type=Parallel  oversample=2  use_embedded=on  pipeline=on  use_rpm=on  placement_style=Rectangular Shape  gen_core=off
      settings: xl_area=[0, 0, 0, 0, 0, 0, 0]
  Mux : xbsIndex_r3/Mux  inputs=3  precision=Full  arith_type="Signed  (2's comp)"  n_bits=8  bin_pt=2  quantization=Truncate  overflow=Wrap  latency=0  explicit_period=off  period=1  en=off  dbl_ovrd=off  show_param=off  mux_type=off  use_rpm=off  gen_core=off
      settings: xl_area=[0, 0, 0, 0, 0, 0, 0]
  Mux1 : xbsIndex_r3/Mux  inputs=3  precision=Full  arith_type="Signed  (2's comp)"  n_bits=8  bin_pt=2  quantization=Truncate  overflow=Wrap  latency=0  explicit_period=off  period=1  en=off  dbl_ovrd=off  show_param=off  mux_type=off  use_rpm=off  gen_core=off
      settings: xl_area=[0, 0, 0, 0, 0, 0, 0]
  Reinterpret : xbsIndex_r3/Reinterpret  force_arith_type=on  arith_type="Signed  (2's comp)"  force_bin_pt=on  bin_pt=17  force_valid=on
  Reinterpret1 : xbsIndex_r3/Reinterpret  force_arith_type=on  arith_type="Signed  (2's comp)"  force_bin_pt=on  bin_pt=17  force_valid=on
  Reinterpret2 : xbsIndex_r3/Reinterpret  force_arith_type=on  arith_type=Unsigned  force_bin_pt=on  bin_pt=0  force_valid=on
  Reinterpret3 : xbsIndex_r3/Reinterpret  force_arith_type=on  arith_type=Unsigned  force_bin_pt=on  bin_pt=0  force_valid=on
  Relational : xbsIndex_r3/Relational  mode=a>b  latency=2  explicit_period=off  period=1  en=off  dbl_ovrd=off  show_param=off
      settings: xl_area=[0, 0, 0, 0, 0, 0, 0]
  Relational1 : xbsIndex_r3/Relational  mode=a<b  latency=2  explicit_period=off  period=1  en=off  dbl_ovrd=off  show_param=off
      settings: xl_area=[0, 0, 0, 0, 0, 0, 0]
  Relational2 : xbsIndex_r3/Relational  mode=a>b  latency=2  explicit_period=off  period=1  en=off  dbl_ovrd=off  show_param=off
      settings: xl_area=[0, 0, 0, 0, 0, 0, 0]
  Relational3 : xbsIndex_r3/Relational  mode=a<b  latency=2  explicit_period=off  period=1  en=off  dbl_ovrd=off  show_param=off
      settings: xl_area=[0, 0, 0, 0, 0, 0, 0]
  Slice4 : xbsIndex_r3/Slice  mode=Upper Bit Location + Width  nbits=18  bit1=0  base1=MSB of Input  bit0=0  base0=LSB of Input  boolean_output=off  explicit_period=off  period=1  dbl_ovrd=off
  Slice5 : xbsIndex_r3/Slice  mode=Lower Bit Location + Width  nbits=18  bit1=0  base1=MSB of Input  bit0=0  base0=LSB of Input  boolean_output=off  explicit_period=off  period=1  dbl_ovrd=off
  dout : Outport
  clip : Outport  Port=2
  wires:
  Logical1/1 -> clip/1
  Mult/1 -> Relational1/1, Relational/1, Convert2/1
  Mult1/1 -> Relational3/1, Relational2/1, Convert3/1
  Mux1/1 -> Reinterpret3/1
  Mux/1 -> Reinterpret2/1
  Relational3/1 -> Logical1/3, Concat2/1
  Relational2/1 -> Logical1/4, Concat2/2
  Constant7/1 -> Mux1/4
  Constant6/1 -> Mux1/3
  Constant5/1 -> Relational3/2
  Constant4/1 -> Relational2/2
  Concat2/1 -> Mux1/1
  Convert3/1 -> Mux1/2
  Relational1/1 -> Logical1/2, Concat1/1
  Relational/1 -> Logical1/1, Concat1/2
  Constant3/1 -> Mux/4
  Constant2/1 -> Mux/3
  Constant1/1 -> Relational1/2
  Constant/1 -> Relational/2
  Concat1/1 -> Mux/1
  Convert2/1 -> Mux/2
  scale/1 -> Mult/2, Mult1/2
  Reinterpret/1 -> Mult/1
  Reinterpret1/1 -> Mult1/1
  Concat/1 -> dout/1
  din/1 -> Slice5/1, Slice4/1
  Reinterpret3/1 -> Concat/2
  Slice5/1 -> Reinterpret1/1
  Reinterpret2/1 -> Concat/1
  Slice4/1 -> Reinterpret/1
